simulink model "FINAL_AUTO_PHASE_2_V4"  (R2020b)
settings: Solver=ode23t  StartTime=0.0  StopTime=180.1  FixedStep=0.05  RelTol=1e-3  EnableMultiTasking=on
model workspace (MAT data in the model file):
  DROP_VACCINE_TIME = 0.25
  GRID_SIDE = 0.457142857143
  HALF_TICKS_TO_DIST = 0.00174532925
  LATCHER_OFFSET = 0.3934603175
  LATCH_CELL_TIME = 0.5
  LOWER_PLATFORM_TIME = 0.5
  NUM_SURVEY_GRIDS = 7
  SPACE_SIDE = 0.152380952381
  SURVEY_GRIDS_CELLS : Simulink.Signal (value not decoded)
  SURVEY_GRIDS_COORDS = [5 5 5 4 5 5 6 6 5 4 3 2 ... (14 elements, 7x2)]
  SURVEY_TURN_ANGLE = 22.7856177106
  WAIT_CONFIRM_CELL_TIME = 0.08
  mapForSim : object (value not decoded)
  occGrid : robotics.BinaryOccupancyGrid (value not decoded)
  oldDetectedCellType : Simulink.Signal (value not decoded)
  unsavedUninfectedCells : Simulink.Signal (value not decoded)
undefined symbols (not defined in the file): cellLevel, cellPose, cellTypeArray, FloorSurface, isoPoses, platformPoses, PlowSurface, Ref, RobotSurface, WallSurface, X, Y, Z
libraries: sm_lib x286, nesl_utility x157, simulink x72, pid_lib x3
(part 14 of 15)

== matlab function FINAL_AUTO_PHASE_2_V4/BEST Robotics 2020 Game (Double-Click)/Cells/Object3/MATLAB Function ==
  settings: updateMethod=DISCRETE
  data: latch input; scoreLevel input; inuse input; target input; time input; objPoseX output; robotPoseX input; robotPoseY input; objPoseY output; latched output; initPose parameter; objId parameter; cellType output; endType output; cellTypeArray parameter; gameTime parameter; platformPoses parameter; cellLevel parameter
function [objPoseX, objPoseY, latched, cellType,endType] = latchObject(latch,scoreLevel, inuse, target, time, robotPoseX, robotPoseY, initPose, objId, cellTypeArray, gameTime, platformPoses, cellLevel)
persistent stateX stateY level pickup
if isempty(stateX)
    stateX=initPose(1);
    stateY=initPose(2);
    level=cellLevel;
    pickup=0;
end

if ~latch
     pickup=0;
    if level && ((stateX > platformPoses(1,1)-0.21 && stateX < platformPoses(1,1)+0.21...
            && stateY > platformPoses(1,2)-0.21 && stateY < platformPoses(1,2) +0.21) || ...
            (stateX > platformPoses(2,1)-0.21 && stateX < platformPoses(2,1)+0.21...
            && stateY > platformPoses(2,2)-0.21 && stateY < platformPoses(2,2) +0.21))
        latched=0.4;
    else
        level=0;
        latched=0;
    end
elseif pickup
    stateX=robotPoseX;
    stateY=robotPoseY;
    level=scoreLevel;
    latched=0.15 +level*0.4;
elseif ~inuse && latch && target == objId && ...
        sqrt((stateX-robotPoseX)^2+(stateY-robotPoseY)^2) < 0.08 && scoreLevel==level
    
        pickup=1;
        latched=0.15;
else
   if level && ((stateX > platformPoses(1,1)-0.21 && stateX < platformPoses(1,1)+0.21...
            && stateY > platformPoses(1,2)-0.21 && stateY < platformPoses(1,2) +0.21) || ...
            (stateX > platformPoses(2,1)-0.21 && stateX < platformPoses(2,1)+0.21...
            && stateY > platformPoses(2,2)-0.21 && stateY < platformPoses(2,2) +0.21))
        latched=0.4;
    else
        level=0;
        latched=0;
    end
end
if sqrt((stateX-robotPoseX)^2+(stateY-robotPoseY)^2) < 0.1 && scoreLevel==level
    cellType=cellTypeArray(objId);
else
    cellType=nan;
end

if time > gameTime
    endType=cellTypeArray(objId)+1;
else
    endType=0;
end

objPoseX=stateX;
objPoseY=stateY;

== matlab function FINAL_AUTO_PHASE_2_V4/BEST Robotics 2020 Game (Double-Click)/Cells/MATLAB Function ==
  data: input input; output output
function output = fcn(input)
output=nan;

for i=1:length(input)
    if ~isnan(input(i))
        output=input(i);
    end
end

== matlab function FINAL_AUTO_PHASE_2_V4/BEST Robotics 2020 Game (Double-Click)/Cells/Object4/MATLAB Function ==
  settings: updateMethod=DISCRETE
  data: latch input; scoreLevel input; inuse input; target input; time input; objPoseX output; robotPoseX input; robotPoseY input; objPoseY output; latched output; initPose parameter; objId parameter; cellType output; endType output; cellTypeArray parameter; gameTime parameter; platformPoses parameter; cellLevel parameter
function [objPoseX, objPoseY, latched, cellType,endType] = latchObject(latch,scoreLevel, inuse, target, time, robotPoseX, robotPoseY, initPose, objId, cellTypeArray, gameTime, platformPoses, cellLevel)
persistent stateX stateY level pickup
if isempty(stateX)
    stateX=initPose(1);
    stateY=initPose(2);
    level=cellLevel;
    pickup=0;
end

if ~latch
     pickup=0;
    if level && ((stateX > platformPoses(1,1)-0.21 && stateX < platformPoses(1,1)+0.21...
            && stateY > platformPoses(1,2)-0.21 && stateY < platformPoses(1,2) +0.21) || ...
            (stateX > platformPoses(2,1)-0.21 && stateX < platformPoses(2,1)+0.21...
            && stateY > platformPoses(2,2)-0.21 && stateY < platformPoses(2,2) +0.21))
        latched=0.4;
    else
        level=0;
        latched=0;
    end
elseif pickup
    stateX=robotPoseX;
    stateY=robotPoseY;
    level=scoreLevel;
    latched=0.15 +level*0.4;
elseif ~inuse && latch && target == objId && ...
        sqrt((stateX-robotPoseX)^2+(stateY-robotPoseY)^2) < 0.08 && scoreLevel==level
    
        pickup=1;
        latched=0.15;
else
   if level && ((stateX > platformPoses(1,1)-0.21 && stateX < platformPoses(1,1)+0.21...
            && stateY > platformPoses(1,2)-0.21 && stateY < platformPoses(1,2) +0.21) || ...
            (stateX > platformPoses(2,1)-0.21 && stateX < platformPoses(2,1)+0.21...
            && stateY > platformPoses(2,2)-0.21 && stateY < platformPoses(2,2) +0.21))
        latched=0.4;
    else
        level=0;
        latched=0;
    end
end
if sqrt((stateX-robotPoseX)^2+(stateY-robotPoseY)^2) < 0.1 && scoreLevel==level
    cellType=cellTypeArray(objId);
else
    cellType=nan;
end

if time > gameTime
    endType=cellTypeArray(objId)+1;
else
    endType=0;
end

objPoseX=stateX;
objPoseY=stateY;

== matlab function FINAL_AUTO_PHASE_2_V4/BEST Robotics 2020 Game (Double-Click)/Cells/Object5/MATLAB Function ==
  settings: updateMethod=DISCRETE
  data: latch input; scoreLevel input; inuse input; target input; time input; objPoseX output; robotPoseX input; robotPoseY input; objPoseY output; latched output; initPose parameter; objId parameter; cellType output; endType output; cellTypeArray parameter; gameTime parameter; platformPoses parameter; cellLevel parameter
function [objPoseX, objPoseY, latched, cellType,endType] = latchObject(latch,scoreLevel, inuse, target, time, robotPoseX, robotPoseY, initPose, objId, cellTypeArray, gameTime, platformPoses, cellLevel)
persistent stateX stateY level pickup
if isempty(stateX)
    stateX=initPose(1);
    stateY=initPose(2);
    level=cellLevel;
    pickup=0;
end

if ~latch
     pickup=0;
    if level && ((stateX > platformPoses(1,1)-0.21 && stateX < platformPoses(1,1)+0.21...
            && stateY > platformPoses(1,2)-0.21 && stateY < platformPoses(1,2) +0.21) || ...
            (stateX > platformPoses(2,1)-0.21 && stateX < platformPoses(2,1)+0.21...
            && stateY > platformPoses(2,2)-0.21 && stateY < platformPoses(2,2) +0.21))
        latched=0.4;
    else
        level=0;
        latched=0;
    end
elseif pickup
    stateX=robotPoseX;
    stateY=robotPoseY;
    level=scoreLevel;
    latched=0.15 +level*0.4;
elseif ~inuse && latch && target == objId && ...
        sqrt((stateX-robotPoseX)^2+(stateY-robotPoseY)^2) < 0.08 && scoreLevel==level
    
        pickup=1;
        latched=0.15;
else
   if level && ((stateX > platformPoses(1,1)-0.21 && stateX < platformPoses(1,1)+0.21...
            && stateY > platformPoses(1,2)-0.21 && stateY < platformPoses(1,2) +0.21) || ...
            (stateX > platformPoses(2,1)-0.21 && stateX < platformPoses(2,1)+0.21...
            && stateY > platformPoses(2,2)-0.21 && stateY < platformPoses(2,2) +0.21))
        latched=0.4;
    else
        level=0;
        latched=0;
    end
end
if sqrt((stateX-robotPoseX)^2+(stateY-robotPoseY)^2) < 0.1 && scoreLevel==level
    cellType=cellTypeArray(objId);
else
    cellType=nan;
end

if time > gameTime
    endType=cellTypeArray(objId)+1;
else
    endType=0;
end

objPoseX=stateX;
objPoseY=stateY;

== matlab function FINAL_AUTO_PHASE_2_V4/BEST Robotics 2020 Game (Double-Click)/Cells/Object1/MATLAB Function ==
  settings: updateMethod=DISCRETE
  data: latch input; scoreLevel input; inuse input; target input; time input; objPoseX output; robotPoseX input; robotPoseY input; objPoseY output; latched output; initPose parameter; objId parameter; cellType output; endType output; cellTypeArray parameter; gameTime parameter; platformPoses parameter; cellLevel parameter
function [objPoseX, objPoseY, latched, cellType,endType] = latchObject(latch,scoreLevel, inuse, target, time, robotPoseX, robotPoseY, initPose, objId, cellTypeArray, gameTime, platformPoses, cellLevel)
persistent stateX stateY level pickup
if isempty(stateX)
    stateX=initPose(1);
    stateY=initPose(2);
    level=cellLevel;
    pickup=0;
end

if ~latch
     pickup=0;
    if level && ((stateX > platformPoses(1,1)-0.21 && stateX < platformPoses(1,1)+0.21...
            && stateY > platformPoses(1,2)-0.21 && stateY < platformPoses(1,2) +0.21) || ...
            (stateX > platformPoses(2,1)-0.21 && stateX < platformPoses(2,1)+0.21...
            && stateY > platformPoses(2,2)-0.21 && stateY < platformPoses(2,2) +0.21))
        latched=0.4;
    else
        level=0;
        latched=0;
    end
elseif pickup
    stateX=robotPoseX;
    stateY=robotPoseY;
    level=scoreLevel;
    latched=0.15 +level*0.4;
elseif ~inuse && latch && target == objId && ...
        sqrt((stateX-robotPoseX)^2+(stateY-robotPoseY)^2) < 0.08 && scoreLevel==level
    
        pickup=1;
        latched=0.15;
else
   if level && ((stateX > platformPoses(1,1)-0.21 && stateX < platformPoses(1,1)+0.21...
            && stateY > platformPoses(1,2)-0.21 && stateY < platformPoses(1,2) +0.21) || ...
            (stateX > platformPoses(2,1)-0.21 && stateX < platformPoses(2,1)+0.21...
            && stateY > platformPoses(2,2)-0.21 && stateY < platformPoses(2,2) +0.21))
        latched=0.4;
    else
        level=0;
        latched=0;
    end
end
if sqrt((stateX-robotPoseX)^2+(stateY-robotPoseY)^2) < 0.1 && scoreLevel==level
    cellType=cellTypeArray(objId);
else
    cellType=nan;
end

if time > gameTime
    endType=cellTypeArray(objId)+1;
else
    endType=0;
end

objPoseX=stateX;
objPoseY=stateY;

== matlab function FINAL_AUTO_PHASE_2_V4/BEST Robotics 2020 Game (Double-Click)/Cells/Object6/MATLAB Function ==
  settings: updateMethod=DISCRETE
  data: latch input; scoreLevel input; inuse input; target input; time input; objPoseX output; robotPoseX input; robotPoseY input; objPoseY output; latched output; initPose parameter; objId parameter; cellType output; endType output; cellTypeArray parameter; gameTime parameter; platformPoses parameter; cellLevel parameter
function [objPoseX, objPoseY, latched, cellType,endType] = latchObject(latch,scoreLevel, inuse, target, time, robotPoseX, robotPoseY, initPose, objId, cellTypeArray, gameTime, platformPoses, cellLevel)
persistent stateX stateY level pickup
if isempty(stateX)
    stateX=initPose(1);
    stateY=initPose(2);
    level=cellLevel;
    pickup=0;
end

if ~latch
     pickup=0;
    if level && ((stateX > platformPoses(1,1)-0.21 && stateX < platformPoses(1,1)+0.21...
            && stateY > platformPoses(1,2)-0.21 && stateY < platformPoses(1,2) +0.21) || ...
            (stateX > platformPoses(2,1)-0.21 && stateX < platformPoses(2,1)+0.21...
            && stateY > platformPoses(2,2)-0.21 && stateY < platformPoses(2,2) +0.21))
        latched=0.4;
    else
        level=0;
        latched=0;
    end
elseif pickup
    stateX=robotPoseX;
    stateY=robotPoseY;
    level=scoreLevel;
    latched=0.15 +level*0.4;
elseif ~inuse && latch && target == objId && ...
        sqrt((stateX-robotPoseX)^2+(stateY-robotPoseY)^2) < 0.08 && scoreLevel==level
    
        pickup=1;
        latched=0.15;
else
   if level && ((stateX > platformPoses(1,1)-0.21 && stateX < platformPoses(1,1)+0.21...
            && stateY > platformPoses(1,2)-0.21 && stateY < platformPoses(1,2) +0.21) || ...
            (stateX > platformPoses(2,1)-0.21 && stateX < platformPoses(2,1)+0.21...
            && stateY > platformPoses(2,2)-0.21 && stateY < platformPoses(2,2) +0.21))
        latched=0.4;
    else
        level=0;
        latched=0;
    end
end
if sqrt((stateX-robotPoseX)^2+(stateY-robotPoseY)^2) < 0.1 && scoreLevel==level
    cellType=cellTypeArray(objId);
else
    cellType=nan;
end

if time > gameTime
    endType=cellTypeArray(objId)+1;
else
    endType=0;
end

objPoseX=stateX;
objPoseY=stateY;

== matlab function FINAL_AUTO_PHASE_2_V4/BEST Robotics 2020 Game (Double-Click)/Cells/Object7/MATLAB Function ==
  settings: updateMethod=DISCRETE
  data: latch input; scoreLevel input; inuse input; target input; time input; objPoseX output; robotPoseX input; robotPoseY input; objPoseY output; latched output; initPose parameter; objId parameter; cellType output; endType output; cellTypeArray parameter; gameTime parameter; platformPoses parameter; cellLevel parameter
function [objPoseX, objPoseY, latched, cellType,endType] = latchObject(latch,scoreLevel, inuse, target, time, robotPoseX, robotPoseY, initPose, objId, cellTypeArray, gameTime, platformPoses, cellLevel)
persistent stateX stateY level pickup
if isempty(stateX)
    stateX=initPose(1);
    stateY=initPose(2);
    level=cellLevel;
    pickup=0;
end

if ~latch
     pickup=0;
    if level && ((stateX > platformPoses(1,1)-0.21 && stateX < platformPoses(1,1)+0.21...
            && stateY > platformPoses(1,2)-0.21 && stateY < platformPoses(1,2) +0.21) || ...
            (stateX > platformPoses(2,1)-0.21 && stateX < platformPoses(2,1)+0.21...
            && stateY > platformPoses(2,2)-0.21 && stateY < platformPoses(2,2) +0.21))
        latched=0.4;
    else
        level=0;
        latched=0;
    end
elseif pickup
    stateX=robotPoseX;
    stateY=robotPoseY;
    level=scoreLevel;
    latched=0.15 +level*0.4;
elseif ~inuse && latch && target == objId && ...
        sqrt((stateX-robotPoseX)^2+(stateY-robotPoseY)^2) < 0.08 && scoreLevel==level
    
        pickup=1;
        latched=0.15;
else
   if level && ((stateX > platformPoses(1,1)-0.21 && stateX < platformPoses(1,1)+0.21...
            && stateY > platformPoses(1,2)-0.21 && stateY < platformPoses(1,2) +0.21) || ...
            (stateX > platformPoses(2,1)-0.21 && stateX < platformPoses(2,1)+0.21...
            && stateY > platformPoses(2,2)-0.21 && stateY < platformPoses(2,2) +0.21))
        latched=0.4;
    else
        level=0;
        latched=0;
    end
end
if sqrt((stateX-robotPoseX)^2+(stateY-robotPoseY)^2) < 0.1 && scoreLevel==level
    cellType=cellTypeArray(objId);
else
    cellType=nan;
end

if time > gameTime
    endType=cellTypeArray(objId)+1;
else
    endType=0;
end

objPoseX=stateX;
objPoseY=stateY;

== matlab function FINAL_AUTO_PHASE_2_V4/BEST Robotics 2020 Game (Double-Click)/Cells/Object8/MATLAB Function ==
  settings: updateMethod=DISCRETE
  data: latch input; scoreLevel input; inuse input; target input; time input; objPoseX output; robotPoseX input; robotPoseY input; objPoseY output; latched output; initPose parameter; objId parameter; cellType output; endType output; cellTypeArray parameter; gameTime parameter; platformPoses parameter; cellLevel parameter
function [objPoseX, objPoseY, latched, cellType,endType] = latchObject(latch,scoreLevel, inuse, target, time, robotPoseX, robotPoseY, initPose, objId, cellTypeArray, gameTime, platformPoses, cellLevel)
persistent stateX stateY level pickup
if isempty(stateX)
    stateX=initPose(1);
    stateY=initPose(2);
    level=cellLevel;
    pickup=0;
end

if ~latch
     pickup=0;
    if level && ((stateX > platformPoses(1,1)-0.21 && stateX < platformPoses(1,1)+0.21...
            && stateY > platformPoses(1,2)-0.21 && stateY < platformPoses(1,2) +0.21) || ...
            (stateX > platformPoses(2,1)-0.21 && stateX < platformPoses(2,1)+0.21...
            && stateY > platformPoses(2,2)-0.21 && stateY < platformPoses(2,2) +0.21))
        latched=0.4;
    else
        level=0;
        latched=0;
    end
elseif pickup
    stateX=robotPoseX;
    stateY=robotPoseY;
    level=scoreLevel;
    latched=0.15 +level*0.4;
elseif ~inuse && latch && target == objId && ...
        sqrt((stateX-robotPoseX)^2+(stateY-robotPoseY)^2) < 0.08 && scoreLevel==level
    
        pickup=1;
        latched=0.15;
else
   if level && ((stateX > platformPoses(1,1)-0.21 && stateX < platformPoses(1,1)+0.21...
            && stateY > platformPoses(1,2)-0.21 && stateY < platformPoses(1,2) +0.21) || ...
            (stateX > platformPoses(2,1)-0.21 && stateX < platformPoses(2,1)+0.21...
            && stateY > platformPoses(2,2)-0.21 && stateY < platformPoses(2,2) +0.21))
        latched=0.4;
    else
        level=0;
        latched=0;
    end
end
if sqrt((stateX-robotPoseX)^2+(stateY-robotPoseY)^2) < 0.1 && scoreLevel==level
    cellType=cellTypeArray(objId);
else
    cellType=nan;
end

if time > gameTime
    endType=cellTypeArray(objId)+1;
else
    endType=0;
end

objPoseX=stateX;
objPoseY=stateY;

== matlab function FINAL_AUTO_PHASE_2_V4/BEST Robotics 2020 Game (Double-Click)/Cells/Object9/MATLAB Function ==
  settings: updateMethod=DISCRETE
  data: latch input; scoreLevel input; inuse input; target input; time input; objPoseX output; robotPoseX input; robotPoseY input; objPoseY output; latched output; initPose parameter; objId parameter; cellType output; endType output; cellTypeArray parameter; gameTime parameter; platformPoses parameter; cellLevel parameter
function [objPoseX, objPoseY, latched, cellType,endType] = latchObject(latch,scoreLevel, inuse, target, time, robotPoseX, robotPoseY, initPose, objId, cellTypeArray, gameTime, platformPoses, cellLevel)
persistent stateX stateY level pickup
if isempty(stateX)
    stateX=initPose(1);
    stateY=initPose(2);
    level=cellLevel;
    pickup=0;
end

if ~latch
     pickup=0;
    if level && ((stateX > platformPoses(1,1)-0.21 && stateX < platformPoses(1,1)+0.21...
            && stateY > platformPoses(1,2)-0.21 && stateY < platformPoses(1,2) +0.21) || ...
            (stateX > platformPoses(2,1)-0.21 && stateX < platformPoses(2,1)+0.21...
            && stateY > platformPoses(2,2)-0.21 && stateY < platformPoses(2,2) +0.21))
        latched=0.4;
    else
        level=0;
        latched=0;
    end
elseif pickup
    stateX=robotPoseX;
    stateY=robotPoseY;
    level=scoreLevel;
    latched=0.15 +level*0.4;
elseif ~inuse && latch && target == objId && ...
        sqrt((stateX-robotPoseX)^2+(stateY-robotPoseY)^2) < 0.08 && scoreLevel==level
    
        pickup=1;
        latched=0.15;
else
   if level && ((stateX > platformPoses(1,1)-0.21 && stateX < platformPoses(1,1)+0.21...
            && stateY > platformPoses(1,2)-0.21 && stateY < platformPoses(1,2) +0.21) || ...
            (stateX > platformPoses(2,1)-0.21 && stateX < platformPoses(2,1)+0.21...
            && stateY > platformPoses(2,2)-0.21 && stateY < platformPoses(2,2) +0.21))
        latched=0.4;
    else
        level=0;
        latched=0;
    end
end
if sqrt((stateX-robotPoseX)^2+(stateY-robotPoseY)^2) < 0.1 && scoreLevel==level
    cellType=cellTypeArray(objId);
else
    cellType=nan;
end

if time > gameTime
    endType=cellTypeArray(objId)+1;
else
    endType=0;
end

objPoseX=stateX;
objPoseY=stateY;

== stateflow chart FINAL_AUTO_PHASE_2_V4/stateflow MAIN_PROGRAM/MAIN_PROGRAM.hasClearedPlatformAt/stateflow hasClearedPlatformAt ==
  state RAISE_LATCHER
    onlyTrackUninfectedCells = false
    platformCleared = false
    entry:
    scoringLevel = 1
  state SURVEY_SEARCH_CELL
  state PLATFORM_CELL_FOUND
    entry:
    leftMotor = 0
    rightMotor = 0
    latchCell = 1
  state LOWER_LATCHER
    entry:
    scoringLevel = 0
  state DROP_CELL
    entry:
    latchCell = 0
    platformCleared = true
  (default) -> RAISE_LATCHER
  DROP_CELL -> RAISE_LATCHER
  RAISE_LATCHER -> SURVEY_SEARCH_CELL : [after(0.25, sec)]
  SURVEY_SEARCH_CELL -> PLATFORM_CELL_FOUND : [surveySweepHasFoundCell(gridX, gridY, false)]
  (default) -> ? [commented out]
  PLATFORM_CELL_FOUND -> LOWER_LATCHER : [after(LATCH_CELL_TIME, sec)]
  LOWER_LATCHER -> DROP_CELL : [after(LOWER_PLATFORM_TIME, sec)]
  data: gridX input; gridY input; scoringLevel data_store_memory; platformCleared output; latchCell data_store_memory; leftMotor data_store_memory; rightMotor data_store_memory; LATCH_CELL_TIME parameter; LOWER_PLATFORM_TIME parameter; onlyTrackUninfectedCells data_store_memory

== stateflow chart FINAL_AUTO_PHASE_2_V4/function hasTurnedToAngle/stateflow postSettleAngle ==
  state SETTLE
  state RESET_MOTORS
    entry:
    leftMotor = 0
    rightMotor = 0
  (default) -> SETTLE
  RESET_MOTORS -> SETTLE
  SETTLE -> RESET_MOTORS : [angleHasSettled]
  data: angleHasSettled input; leftMotor data_store_memory; rightMotor data_store_memory

== matlab function FINAL_AUTO_PHASE_2_V4/BEST Robotics 2020 Game (Double-Click)/Cells/Object10/MATLAB Function ==
  settings: updateMethod=DISCRETE
  data: latch input; scoreLevel input; inuse input; target input; time input; objPoseX output; robotPoseX input; robotPoseY input; objPoseY output; latched output; initPose parameter; objId parameter; cellType output; endType output; cellTypeArray parameter; gameTime parameter; platformPoses parameter; cellLevel parameter
function [objPoseX, objPoseY, latched, cellType,endType] = latchObject(latch,scoreLevel, inuse, target, time, robotPoseX, robotPoseY, initPose, objId, cellTypeArray, gameTime, platformPoses, cellLevel)
persistent stateX stateY level pickup
if isempty(stateX)
    stateX=initPose(1);
    stateY=initPose(2);
    level=cellLevel;
    pickup=0;
end

if ~latch
     pickup=0;
    if level && ((stateX > platformPoses(1,1)-0.21 && stateX < platformPoses(1,1)+0.21...
            && stateY > platformPoses(1,2)-0.21 && stateY < platformPoses(1,2) +0.21) || ...
            (stateX > platformPoses(2,1)-0.21 && stateX < platformPoses(2,1)+0.21...
            && stateY > platformPoses(2,2)-0.21 && stateY < platformPoses(2,2) +0.21))
        latched=0.4;
    else
        level=0;
        latched=0;
    end
elseif pickup
    stateX=robotPoseX;
    stateY=robotPoseY;
    level=scoreLevel;
    latched=0.15 +level*0.4;
elseif ~inuse && latch && target == objId && ...
        sqrt((stateX-robotPoseX)^2+(stateY-robotPoseY)^2) < 0.08 && scoreLevel==level
    
        pickup=1;
        latched=0.15;
else
   if level && ((stateX > platformPoses(1,1)-0.21 && stateX < platformPoses(1,1)+0.21...
            && stateY > platformPoses(1,2)-0.21 && stateY < platformPoses(1,2) +0.21) || ...
            (stateX > platformPoses(2,1)-0.21 && stateX < platformPoses(2,1)+0.21...
            && stateY > platformPoses(2,2)-0.21 && stateY < platformPoses(2,2) +0.21))
        latched=0.4;
    else
        level=0;
        latched=0;
    end
end
if sqrt((stateX-robotPoseX)^2+(stateY-robotPoseY)^2) < 0.1 && scoreLevel==level
    cellType=cellTypeArray(objId);
else
    cellType=nan;
end

if time > gameTime
    endType=cellTypeArray(objId)+1;
else
    endType=0;
end

objPoseX=stateX;
objPoseY=stateY;

== matlab function FINAL_AUTO_PHASE_2_V4/BEST Robotics 2020 Game (Double-Click)/Cells/Object11/MATLAB Function ==
  settings: updateMethod=DISCRETE
  data: latch input; scoreLevel input; inuse input; target input; time input; objPoseX output; robotPoseX input; robotPoseY input; objPoseY output; latched output; initPose parameter; objId parameter; cellType output; endType output; cellTypeArray parameter; gameTime parameter; platformPoses parameter; cellLevel parameter
function [objPoseX, objPoseY, latched, cellType,endType] = latchObject(latch,scoreLevel, inuse, target, time, robotPoseX, robotPoseY, initPose, objId, cellTypeArray, gameTime, platformPoses, cellLevel)
persistent stateX stateY level pickup
if isempty(stateX)
    stateX=initPose(1);
    stateY=initPose(2);
    level=cellLevel;
    pickup=0;
end

if ~latch
     pickup=0;
    if level && ((stateX > platformPoses(1,1)-0.21 && stateX < platformPoses(1,1)+0.21...
            && stateY > platformPoses(1,2)-0.21 && stateY < platformPoses(1,2) +0.21) || ...
            (stateX > platformPoses(2,1)-0.21 && stateX < platformPoses(2,1)+0.21...
            && stateY > platformPoses(2,2)-0.21 && stateY < platformPoses(2,2) +0.21))
        latched=0.4;
    else
        level=0;
        latched=0;
    end
elseif pickup
    stateX=robotPoseX;
    stateY=robotPoseY;
    level=scoreLevel;
    latched=0.15 +level*0.4;
elseif ~inuse && latch && target == objId && ...
        sqrt((stateX-robotPoseX)^2+(stateY-robotPoseY)^2) < 0.08 && scoreLevel==level
    
        pickup=1;
        latched=0.15;
else
   if level && ((stateX > platformPoses(1,1)-0.21 && stateX < platformPoses(1,1)+0.21...
            && stateY > platformPoses(1,2)-0.21 && stateY < platformPoses(1,2) +0.21) || ...
            (stateX > platformPoses(2,1)-0.21 && stateX < platformPoses(2,1)+0.21...
            && stateY > platformPoses(2,2)-0.21 && stateY < platformPoses(2,2) +0.21))
        latched=0.4;
    else
        level=0;
        latched=0;
    end
end
if sqrt((stateX-robotPoseX)^2+(stateY-robotPoseY)^2) < 0.1 && scoreLevel==level
    cellType=cellTypeArray(objId);
else
    cellType=nan;
end

if time > gameTime
    endType=cellTypeArray(objId)+1;
else
    endType=0;
end

objPoseX=stateX;
objPoseY=stateY;

== matlab function FINAL_AUTO_PHASE_2_V4/BEST Robotics 2020 Game (Double-Click)/Cells/Object12/MATLAB Function ==
  settings: updateMethod=DISCRETE
  data: latch input; scoreLevel input; inuse input; target input; time input; objPoseX output; robotPoseX input; robotPoseY input; objPoseY output; latched output; initPose parameter; objId parameter; cellType output; endType output; cellTypeArray parameter; gameTime parameter; platformPoses parameter; cellLevel parameter
function [objPoseX, objPoseY, latched, cellType,endType] = latchObject(latch,scoreLevel, inuse, target, time, robotPoseX, robotPoseY, initPose, objId, cellTypeArray, gameTime, platformPoses, cellLevel)
persistent stateX stateY level pickup
if isempty(stateX)
    stateX=initPose(1);
    stateY=initPose(2);
    level=cellLevel;
    pickup=0;
end

if ~latch
     pickup=0;
    if level && ((stateX > platformPoses(1,1)-0.21 && stateX < platformPoses(1,1)+0.21...
            && stateY > platformPoses(1,2)-0.21 && stateY < platformPoses(1,2) +0.21) || ...
            (stateX > platformPoses(2,1)-0.21 && stateX < platformPoses(2,1)+0.21...
            && stateY > platformPoses(2,2)-0.21 && stateY < platformPoses(2,2) +0.21))
        latched=0.4;
    else
        level=0;
        latched=0;
    end
elseif pickup
    stateX=robotPoseX;
    stateY=robotPoseY;
    level=scoreLevel;
    latched=0.15 +level*0.4;
elseif ~inuse && latch && target == objId && ...
        sqrt((stateX-robotPoseX)^2+(stateY-robotPoseY)^2) < 0.08 && scoreLevel==level
    
        pickup=1;
        latched=0.15;
else
   if level && ((stateX > platformPoses(1,1)-0.21 && stateX < platformPoses(1,1)+0.21...
            && stateY > platformPoses(1,2)-0.21 && stateY < platformPoses(1,2) +0.21) || ...
            (stateX > platformPoses(2,1)-0.21 && stateX < platformPoses(2,1)+0.21...
            && stateY > platformPoses(2,2)-0.21 && stateY < platformPoses(2,2) +0.21))
        latched=0.4;
    else
        level=0;
        latched=0;
    end
end
if sqrt((stateX-robotPoseX)^2+(stateY-robotPoseY)^2) < 0.1 && scoreLevel==level
    cellType=cellTypeArray(objId);
else
    cellType=nan;
end

if time > gameTime
    endType=cellTypeArray(objId)+1;
else
    endType=0;
end

objPoseX=stateX;
objPoseY=stateY;

== matlab function FINAL_AUTO_PHASE_2_V4/BEST Robotics 2020 Game (Double-Click)/Cells/Object13/MATLAB Function ==
  settings: updateMethod=DISCRETE
  data: latch input; scoreLevel input; inuse input; target input; time input; objPoseX output; robotPoseX input; robotPoseY input; objPoseY output; latched output; initPose parameter; objId parameter; cellType output; endType output; cellTypeArray parameter; gameTime parameter; platformPoses parameter; cellLevel parameter
function [objPoseX, objPoseY, latched, cellType,endType] = latchObject(latch,scoreLevel, inuse, target, time, robotPoseX, robotPoseY, initPose, objId, cellTypeArray, gameTime, platformPoses, cellLevel)
persistent stateX stateY level pickup
if isempty(stateX)
    stateX=initPose(1);
    stateY=initPose(2);
    level=cellLevel;
    pickup=0;
end

if ~latch
     pickup=0;
    if level && ((stateX > platformPoses(1,1)-0.21 && stateX < platformPoses(1,1)+0.21...
            && stateY > platformPoses(1,2)-0.21 && stateY < platformPoses(1,2) +0.21) || ...
            (stateX > platformPoses(2,1)-0.21 && stateX < platformPoses(2,1)+0.21...
            && stateY > platformPoses(2,2)-0.21 && stateY < platformPoses(2,2) +0.21))
        latched=0.4;
    else
        level=0;
        latched=0;
    end
elseif pickup
    stateX=robotPoseX;
    stateY=robotPoseY;
    level=scoreLevel;
    latched=0.15 +level*0.4;
elseif ~inuse && latch && target == objId && ...
        sqrt((stateX-robotPoseX)^2+(stateY-robotPoseY)^2) < 0.08 && scoreLevel==level
    
        pickup=1;
        latched=0.15;
else
   if level && ((stateX > platformPoses(1,1)-0.21 && stateX < platformPoses(1,1)+0.21...
            && stateY > platformPoses(1,2)-0.21 && stateY < platformPoses(1,2) +0.21) || ...
            (stateX > platformPoses(2,1)-0.21 && stateX < platformPoses(2,1)+0.21...
            && stateY > platformPoses(2,2)-0.21 && stateY < platformPoses(2,2) +0.21))
        latched=0.4;
    else
        level=0;
        latched=0;
    end
end
if sqrt((stateX-robotPoseX)^2+(stateY-robotPoseY)^2) < 0.1 && scoreLevel==level
    cellType=cellTypeArray(objId);
else
    cellType=nan;
end

if time > gameTime
    endType=cellTypeArray(objId)+1;
else
    endType=0;
end

objPoseX=stateX;
objPoseY=stateY;

== matlab function FINAL_AUTO_PHASE_2_V4/BEST Robotics 2020 Game (Double-Click)/Cells/Object14/MATLAB Function ==
  settings: updateMethod=DISCRETE
  data: latch input; scoreLevel input; inuse input; target input; time input; objPoseX output; robotPoseX input; robotPoseY input; objPoseY output; latched output; initPose parameter; objId parameter; cellType output; endType output; cellTypeArray parameter; gameTime parameter; platformPoses parameter; cellLevel parameter
function [objPoseX, objPoseY, latched, cellType,endType] = latchObject(latch,scoreLevel, inuse, target, time, robotPoseX, robotPoseY, initPose, objId, cellTypeArray, gameTime, platformPoses, cellLevel)
persistent stateX stateY level pickup
if isempty(stateX)
    stateX=initPose(1);
    stateY=initPose(2);
    level=cellLevel;
    pickup=0;
end

if ~latch
     pickup=0;
    if level && ((stateX > platformPoses(1,1)-0.21 && stateX < platformPoses(1,1)+0.21...
            && stateY > platformPoses(1,2)-0.21 && stateY < platformPoses(1,2) +0.21) || ...
            (stateX > platformPoses(2,1)-0.21 && stateX < platformPoses(2,1)+0.21...
            && stateY > platformPoses(2,2)-0.21 && stateY < platformPoses(2,2) +0.21))
        latched=0.4;
    else
        level=0;
        latched=0;
    end
elseif pickup
    stateX=robotPoseX;
    stateY=robotPoseY;
    level=scoreLevel;
    latched=0.15 +level*0.4;
elseif ~inuse && latch && target == objId && ...
        sqrt((stateX-robotPoseX)^2+(stateY-robotPoseY)^2) < 0.08 && scoreLevel==level
    
        pickup=1;
        latched=0.15;
else
   if level && ((stateX > platformPoses(1,1)-0.21 && stateX < platformPoses(1,1)+0.21...
            && stateY > platformPoses(1,2)-0.21 && stateY < platformPoses(1,2) +0.21) || ...
            (stateX > platformPoses(2,1)-0.21 && stateX < platformPoses(2,1)+0.21...
            && stateY > platformPoses(2,2)-0.21 && stateY < platformPoses(2,2) +0.21))
        latched=0.4;
    else
        level=0;
        latched=0;
    end
end
if sqrt((stateX-robotPoseX)^2+(stateY-robotPoseY)^2) < 0.1 && scoreLevel==level
    cellType=cellTypeArray(objId);
else
    cellType=nan;
end

if time > gameTime
    endType=cellTypeArray(objId)+1;
else
    endType=0;
end

objPoseX=stateX;
objPoseY=stateY;

== matlab function FINAL_AUTO_PHASE_2_V4/BEST Robotics 2020 Game (Double-Click)/Cells/Object15/MATLAB Function ==
  settings: updateMethod=DISCRETE
  data: latch input; scoreLevel input; inuse input; target input; time input; objPoseX output; robotPoseX input; robotPoseY input; objPoseY output; latched output; initPose parameter; objId parameter; cellType output; endType output; cellTypeArray parameter; gameTime parameter; platformPoses parameter; cellLevel parameter
function [objPoseX, objPoseY, latched, cellType,endType] = latchObject(latch,scoreLevel, inuse, target, time, robotPoseX, robotPoseY, initPose, objId, cellTypeArray, gameTime, platformPoses, cellLevel)
persistent stateX stateY level pickup
if isempty(stateX)
    stateX=initPose(1);
    stateY=initPose(2);
    level=cellLevel;
    pickup=0;
end

if ~latch
     pickup=0;
    if level && ((stateX > platformPoses(1,1)-0.21 && stateX < platformPoses(1,1)+0.21...
            && stateY > platformPoses(1,2)-0.21 && stateY < platformPoses(1,2) +0.21) || ...
            (stateX > platformPoses(2,1)-0.21 && stateX < platformPoses(2,1)+0.21...
            && stateY > platformPoses(2,2)-0.21 && stateY < platformPoses(2,2) +0.21))
        latched=0.4;
    else
        level=0;
        latched=0;
    end
elseif pickup
    stateX=robotPoseX;
    stateY=robotPoseY;
    level=scoreLevel;
    latched=0.15 +level*0.4;
elseif ~inuse && latch && target == objId && ...
        sqrt((stateX-robotPoseX)^2+(stateY-robotPoseY)^2) < 0.08 && scoreLevel==level
    
        pickup=1;
        latched=0.15;
else
   if level && ((stateX > platformPoses(1,1)-0.21 && stateX < platformPoses(1,1)+0.21...
            && stateY > platformPoses(1,2)-0.21 && stateY < platformPoses(1,2) +0.21) || ...
            (stateX > platformPoses(2,1)-0.21 && stateX < platformPoses(2,1)+0.21...
            && stateY > platformPoses(2,2)-0.21 && stateY < platformPoses(2,2) +0.21))
        latched=0.4;
    else
        level=0;
        latched=0;
    end
end
if sqrt((stateX-robotPoseX)^2+(stateY-robotPoseY)^2) < 0.1 && scoreLevel==level
    cellType=cellTypeArray(objId);
else
    cellType=nan;
end

if time > gameTime
    endType=cellTypeArray(objId)+1;
else
    endType=0;
end

objPoseX=stateX;
objPoseY=stateY;

== matlab function FINAL_AUTO_PHASE_2_V4/BEST Robotics 2020 Game (Double-Click)/Cells/Object16/MATLAB Function ==
  settings: updateMethod=DISCRETE
  data: latch input; scoreLevel input; inuse input; target input; time input; objPoseX output; robotPoseX input; robotPoseY input; objPoseY output; latched output; initPose parameter; objId parameter; cellType output; endType output; cellTypeArray parameter; gameTime parameter; platformPoses parameter; cellLevel parameter
function [objPoseX, objPoseY, latched, cellType,endType] = latchObject(latch,scoreLevel, inuse, target, time, robotPoseX, robotPoseY, initPose, objId, cellTypeArray, gameTime, platformPoses, cellLevel)
persistent stateX stateY level pickup
if isempty(stateX)
    stateX=initPose(1);
    stateY=initPose(2);
    level=cellLevel;
    pickup=0;
end

if ~latch
     pickup=0;
    if level && ((stateX > platformPoses(1,1)-0.21 && stateX < platformPoses(1,1)+0.21...
            && stateY > platformPoses(1,2)-0.21 && stateY < platformPoses(1,2) +0.21) || ...
            (stateX > platformPoses(2,1)-0.21 && stateX < platformPoses(2,1)+0.21...
            && stateY > platformPoses(2,2)-0.21 && stateY < platformPoses(2,2) +0.21))
        latched=0.4;
    else
        level=0;
        latched=0;
    end
elseif pickup
    stateX=robotPoseX;
    stateY=robotPoseY;
    level=scoreLevel;
    latched=0.15 +level*0.4;
elseif ~inuse && latch && target == objId && ...
        sqrt((stateX-robotPoseX)^2+(stateY-robotPoseY)^2) < 0.08 && scoreLevel==level
    
        pickup=1;
        latched=0.15;
else
   if level && ((stateX > platformPoses(1,1)-0.21 && stateX < platformPoses(1,1)+0.21...
            && stateY > platformPoses(1,2)-0.21 && stateY < platformPoses(1,2) +0.21) || ...
            (stateX > platformPoses(2,1)-0.21 && stateX < platformPoses(2,1)+0.21...
            && stateY > platformPoses(2,2)-0.21 && stateY < platformPoses(2,2) +0.21))
        latched=0.4;
    else
        level=0;
        latched=0;
    end
end
if sqrt((stateX-robotPoseX)^2+(stateY-robotPoseY)^2) < 0.1 && scoreLevel==level
    cellType=cellTypeArray(objId);
else
    cellType=nan;
end

if time > gameTime
    endType=cellTypeArray(objId)+1;
else
    endType=0;
end

objPoseX=stateX;
objPoseY=stateY;

== matlab function FINAL_AUTO_PHASE_2_V4/BEST Robotics 2020 Game (Double-Click)/Cells/Object17/MATLAB Function ==
  settings: updateMethod=DISCRETE
  data: latch input; scoreLevel input; inuse input; target input; time input; objPoseX output; robotPoseX input; robotPoseY input; objPoseY output; latched output; initPose parameter; objId parameter; cellType output; endType output; cellTypeArray parameter; gameTime parameter; platformPoses parameter; cellLevel parameter
function [objPoseX, objPoseY, latched, cellType,endType] = latchObject(latch,scoreLevel, inuse, target, time, robotPoseX, robotPoseY, initPose, objId, cellTypeArray, gameTime, platformPoses, cellLevel)
persistent stateX stateY level pickup
if isempty(stateX)
    stateX=initPose(1);
    stateY=initPose(2);
    level=cellLevel;
    pickup=0;
end

if ~latch
     pickup=0;
    if level && ((stateX > platformPoses(1,1)-0.21 && stateX < platformPoses(1,1)+0.21...
            && stateY > platformPoses(1,2)-0.21 && stateY < platformPoses(1,2) +0.21) || ...
            (stateX > platformPoses(2,1)-0.21 && stateX < platformPoses(2,1)+0.21...
            && stateY > platformPoses(2,2)-0.21 && stateY < platformPoses(2,2) +0.21))
        latched=0.4;
    else
        level=0;
        latched=0;
    end
elseif pickup
    stateX=robotPoseX;
    stateY=robotPoseY;
    level=scoreLevel;
    latched=0.15 +level*0.4;
elseif ~inuse && latch && target == objId && ...
        sqrt((stateX-robotPoseX)^2+(stateY-robotPoseY)^2) < 0.08 && scoreLevel==level
    
        pickup=1;
        latched=0.15;
else
   if level && ((stateX > platformPoses(1,1)-0.21 && stateX < platformPoses(1,1)+0.21...
            && stateY > platformPoses(1,2)-0.21 && stateY < platformPoses(1,2) +0.21) || ...
            (stateX > platformPoses(2,1)-0.21 && stateX < platformPoses(2,1)+0.21...
            && stateY > platformPoses(2,2)-0.21 && stateY < platformPoses(2,2) +0.21))
        latched=0.4;
    else
        level=0;
        latched=0;
    end
end
if sqrt((stateX-robotPoseX)^2+(stateY-robotPoseY)^2) < 0.1 && scoreLevel==level
    cellType=cellTypeArray(objId);
else
    cellType=nan;
end

if time > gameTime
    endType=cellTypeArray(objId)+1;
else
    endType=0;
end

objPoseX=stateX;
objPoseY=stateY;

== matlab function FINAL_AUTO_PHASE_2_V4/BEST Robotics 2020 Game (Double-Click)/Cells/Object18/MATLAB Function ==
  settings: updateMethod=DISCRETE
  data: latch input; scoreLevel input; inuse input; target input; time input; objPoseX output; robotPoseX input; robotPoseY input; objPoseY output; latched output; initPose parameter; objId parameter; cellType output; endType output; cellTypeArray parameter; gameTime parameter; platformPoses parameter; cellLevel parameter
function [objPoseX, objPoseY, latched, cellType,endType] = latchObject(latch,scoreLevel, inuse, target, time, robotPoseX, robotPoseY, initPose, objId, cellTypeArray, gameTime, platformPoses, cellLevel)
persistent stateX stateY level pickup
if isempty(stateX)
    stateX=initPose(1);
    stateY=initPose(2);
    level=cellLevel;
    pickup=0;
end

if ~latch
     pickup=0;
    if level && ((stateX > platformPoses(1,1)-0.21 && stateX < platformPoses(1,1)+0.21...
            && stateY > platformPoses(1,2)-0.21 && stateY < platformPoses(1,2) +0.21) || ...
            (stateX > platformPoses(2,1)-0.21 && stateX < platformPoses(2,1)+0.21...
            && stateY > platformPoses(2,2)-0.21 && stateY < platformPoses(2,2) +0.21))
        latched=0.4;
    else
        level=0;
        latched=0;
    end
elseif pickup
    stateX=robotPoseX;
    stateY=robotPoseY;
    level=scoreLevel;
    latched=0.15 +level*0.4;
elseif ~inuse && latch && target == objId && ...
        sqrt((stateX-robotPoseX)^2+(stateY-robotPoseY)^2) < 0.08 && scoreLevel==level
    
        pickup=1;
        latched=0.15;
else
   if level && ((stateX > platformPoses(1,1)-0.21 && stateX < platformPoses(1,1)+0.21...
            && stateY > platformPoses(1,2)-0.21 && stateY < platformPoses(1,2) +0.21) || ...
            (stateX > platformPoses(2,1)-0.21 && stateX < platformPoses(2,1)+0.21...
            && stateY > platformPoses(2,2)-0.21 && stateY < platformPoses(2,2) +0.21))
        latched=0.4;
    else
        level=0;
        latched=0;
    end
end
if sqrt((stateX-robotPoseX)^2+(stateY-robotPoseY)^2) < 0.1 && scoreLevel==level
    cellType=cellTypeArray(objId);
else
    cellType=nan;
end

if time > gameTime
    endType=cellTypeArray(objId)+1;
else
    endType=0;
end

objPoseX=stateX;
objPoseY=stateY;

== matlab function FINAL_AUTO_PHASE_2_V4/BEST Robotics 2020 Game (Double-Click)/Cells/Object19/MATLAB Function ==
  settings: updateMethod=DISCRETE
  data: latch input; scoreLevel input; inuse input; target input; time input; objPoseX output; robotPoseX input; robotPoseY input; objPoseY output; latched output; initPose parameter; objId parameter; cellType output; endType output; cellTypeArray parameter; gameTime parameter; platformPoses parameter; cellLevel parameter
function [objPoseX, objPoseY, latched, cellType,endType] = latchObject(latch,scoreLevel, inuse, target, time, robotPoseX, robotPoseY, initPose, objId, cellTypeArray, gameTime, platformPoses, cellLevel)
persistent stateX stateY level pickup
if isempty(stateX)
    stateX=initPose(1);
    stateY=initPose(2);
    level=cellLevel;
    pickup=0;
end

if ~latch
     pickup=0;
    if level && ((stateX > platformPoses(1,1)-0.21 && stateX < platformPoses(1,1)+0.21...
            && stateY > platformPoses(1,2)-0.21 && stateY < platformPoses(1,2) +0.21) || ...
            (stateX > platformPoses(2,1)-0.21 && stateX < platformPoses(2,1)+0.21...
            && stateY > platformPoses(2,2)-0.21 && stateY < platformPoses(2,2) +0.21))
        latched=0.4;
    else
        level=0;
        latched=0;
    end
elseif pickup
    stateX=robotPoseX;
    stateY=robotPoseY;
    level=scoreLevel;
    latched=0.15 +level*0.4;
elseif ~inuse && latch && target == objId && ...
        sqrt((stateX-robotPoseX)^2+(stateY-robotPoseY)^2) < 0.08 && scoreLevel==level
    
        pickup=1;
        latched=0.15;
else
   if level && ((stateX > platformPoses(1,1)-0.21 && stateX < platformPoses(1,1)+0.21...
            && stateY > platformPoses(1,2)-0.21 && stateY < platformPoses(1,2) +0.21) || ...
            (stateX > platformPoses(2,1)-0.21 && stateX < platformPoses(2,1)+0.21...
            && stateY > platformPoses(2,2)-0.21 && stateY < platformPoses(2,2) +0.21))
        latched=0.4;
    else
        level=0;
        latched=0;
    end
end
if sqrt((stateX-robotPoseX)^2+(stateY-robotPoseY)^2) < 0.1 && scoreLevel==level
    cellType=cellTypeArray(objId);
else
    cellType=nan;
end

if time > gameTime
    endType=cellTypeArray(objId)+1;
else
    endType=0;
end

objPoseX=stateX;
objPoseY=stateY;

== matlab function FINAL_AUTO_PHASE_2_V4/BEST Robotics 2020 Game (Double-Click)/Cells/Object20/MATLAB Function ==
  settings: updateMethod=DISCRETE
  data: latch input; scoreLevel input; inuse input; target input; time input; objPoseX output; robotPoseX input; robotPoseY input; objPoseY output; latched output; initPose parameter; objId parameter; cellType output; endType output; cellTypeArray parameter; gameTime parameter; platformPoses parameter; cellLevel parameter
function [objPoseX, objPoseY, latched, cellType,endType] = latchObject(latch,scoreLevel, inuse, target, time, robotPoseX, robotPoseY, initPose, objId, cellTypeArray, gameTime, platformPoses, cellLevel)
persistent stateX stateY level pickup
if isempty(stateX)
    stateX=initPose(1);
    stateY=initPose(2);
    level=cellLevel;
    pickup=0;
end

if ~latch
     pickup=0;
    if level && ((stateX > platformPoses(1,1)-0.21 && stateX < platformPoses(1,1)+0.21...
            && stateY > platformPoses(1,2)-0.21 && stateY < platformPoses(1,2) +0.21) || ...
            (stateX > platformPoses(2,1)-0.21 && stateX < platformPoses(2,1)+0.21...
            && stateY > platformPoses(2,2)-0.21 && stateY < platformPoses(2,2) +0.21))
        latched=0.4;
    else
        level=0;
        latched=0;
    end
elseif pickup
    stateX=robotPoseX;
    stateY=robotPoseY;
    level=scoreLevel;
    latched=0.15 +level*0.4;
elseif ~inuse && latch && target == objId && ...
        sqrt((stateX-robotPoseX)^2+(stateY-robotPoseY)^2) < 0.08 && scoreLevel==level
    
        pickup=1;
        latched=0.15;
else
   if level && ((stateX > platformPoses(1,1)-0.21 && stateX < platformPoses(1,1)+0.21...
            && stateY > platformPoses(1,2)-0.21 && stateY < platformPoses(1,2) +0.21) || ...
            (stateX > platformPoses(2,1)-0.21 && stateX < platformPoses(2,1)+0.21...
            && stateY > platformPoses(2,2)-0.21 && stateY < platformPoses(2,2) +0.21))
        latched=0.4;
    else
        level=0;
        latched=0;
    end
end
if sqrt((stateX-robotPoseX)^2+(stateY-robotPoseY)^2) < 0.1 && scoreLevel==level
    cellType=cellTypeArray(objId);
else
    cellType=nan;
end

if time > gameTime
    endType=cellTypeArray(objId)+1;
else
    endType=0;
end

objPoseX=stateX;
objPoseY=stateY;

== matlab function FINAL_AUTO_PHASE_2_V4/BEST Robotics 2020 Game (Double-Click)/Cells/Object21/MATLAB Function ==
  settings: updateMethod=DISCRETE
  data: latch input; scoreLevel input; inuse input; target input; time input; objPoseX output; robotPoseX input; robotPoseY input; objPoseY output; latched output; initPose parameter; objId parameter; cellType output; endType output; cellTypeArray parameter; gameTime parameter; platformPoses parameter; cellLevel parameter
function [objPoseX, objPoseY, latched, cellType,endType] = latchObject(latch,scoreLevel, inuse, target, time, robotPoseX, robotPoseY, initPose, objId, cellTypeArray, gameTime, platformPoses, cellLevel)
persistent stateX stateY level pickup
if isempty(stateX)
    stateX=initPose(1);
    stateY=initPose(2);
    level=cellLevel;
    pickup=0;
end

if ~latch
     pickup=0;
    if level && ((stateX > platformPoses(1,1)-0.21 && stateX < platformPoses(1,1)+0.21...
            && stateY > platformPoses(1,2)-0.21 && stateY < platformPoses(1,2) +0.21) || ...
            (stateX > platformPoses(2,1)-0.21 && stateX < platformPoses(2,1)+0.21...
            && stateY > platformPoses(2,2)-0.21 && stateY < platformPoses(2,2) +0.21))
        latched=0.4;
    else
        level=0;
        latched=0;
    end
elseif pickup
    stateX=robotPoseX;
    stateY=robotPoseY;
    level=scoreLevel;
    latched=0.15 +level*0.4;
elseif ~inuse && latch && target == objId && ...
        sqrt((stateX-robotPoseX)^2+(stateY-robotPoseY)^2) < 0.08 && scoreLevel==level
    
        pickup=1;
        latched=0.15;
else
   if level && ((stateX > platformPoses(1,1)-0.21 && stateX < platformPoses(1,1)+0.21...
            && stateY > platformPoses(1,2)-0.21 && stateY < platformPoses(1,2) +0.21) || ...
            (stateX > platformPoses(2,1)-0.21 && stateX < platformPoses(2,1)+0.21...
            && stateY > platformPoses(2,2)-0.21 && stateY < platformPoses(2,2) +0.21))
        latched=0.4;
    else
        level=0;
        latched=0;
    end
end
if sqrt((stateX-robotPoseX)^2+(stateY-robotPoseY)^2) < 0.1 && scoreLevel==level
    cellType=cellTypeArray(objId);
else
    cellType=nan;
end

if time > gameTime
    endType=cellTypeArray(objId)+1;
else
    endType=0;
end

objPoseX=stateX;
objPoseY=stateY;

== matlab function FINAL_AUTO_PHASE_2_V4/BEST Robotics 2020 Game (Double-Click)/Cells/MATLAB Function2 ==
  data: robotPose input; cellPoses input; cellTarget output
function cellTarget = findTarget(robotPose, cellPoses)


eucDist=sqrt((cellPoses(:,1)-robotPose(1)).^2+(cellPoses(:,2)-robotPose(2)).^2);
[~,cellIdx]=min(eucDist);
cellTarget = cellIdx;

== matlab function FINAL_AUTO_PHASE_2_V4/BEST Robotics 2020 Game (Double-Click)/Vaccines/Vaccine/MATLAB Function ==
  settings: updateMethod=DISCRETE
  data: drop input; level input; objPoseX output; robotPoseX input; robotPoseY input; objPoseY output; vaccine output
function [objPoseX, objPoseY, vaccine] = latchObject(drop, level, robotPoseX, robotPoseY)
persistent stateX stateY stateZ prevDrop dropped
if isempty(stateX)
    stateX=robotPoseX+0.14;
    stateY=robotPoseY;
    stateZ=0.15;
    prevDrop=0;
    dropped=0;
end

if drop && prevDrop && ~dropped
    stateX=robotPoseX;
    stateY=robotPoseY;
    stateZ=level*0.4;
    objPoseX=robotPoseX;
    objPoseY=robotPoseY;
    dropped=1;
elseif dropped
    objPoseX=stateX;
    objPoseY=stateY;

else
    objPoseX=robotPoseX+0.14;
    objPoseY=robotPoseY;
end
prevDrop=drop;
vaccine=stateZ;

== matlab function FINAL_AUTO_PHASE_2_V4/BEST Robotics 2020 Game (Double-Click)/Vaccines/Vaccine2/MATLAB Function1 ==
  settings: updateMethod=DISCRETE
  data: drop input; level input; objPoseX output; robotPoseX input; robotPoseY input; objPoseY output; vaccine output
function [objPoseX, objPoseY, vaccine] = latchObject(drop, level, robotPoseX, robotPoseY)
persistent stateX stateY stateZ prevDrop dropped
if isempty(stateX)
    stateX=robotPoseX+0.14;
    stateY=robotPoseY;
    stateZ=0.15;
    prevDrop=0;
    dropped=0;
end

if drop && prevDrop && ~dropped
    stateX=robotPoseX;
    stateY=robotPoseY;
    stateZ=level*0.4;
    objPoseX=robotPoseX;
    objPoseY=robotPoseY;
    dropped=1;
elseif dropped
    objPoseX=stateX;
    objPoseY=stateY;

else
    objPoseX=robotPoseX-0.11;
    objPoseY=robotPoseY+0.11;
end
prevDrop=drop;
vaccine=stateZ;
